simulink library "cyclopsLib"  (R2020a)
settings: Solver=VariableStepAuto  StartTime=0.0  StopTime=10.0  RelTol=1e-3
values from neighbouring files (symbols this model uses):
  agc_delay_lag = 32    [rev0BB_setup.m]
  agc_detector_coef = ones(1,agc_detector_taps)./agc_detector_taps    [rev0BB_setup.m]
  agc_sat_low = -agcSaturation    (= -12)    [rev0BB_setup.m]
  agc_sat_up = agcSaturation    (= 12)    [rev0BB_setup.m]
  agcDesired = 0    [rev0BB_setup.m]
  agcExpDomain = agcSaturation    (= 12)    [rev0BB_setup.m]
  agcExpResolution = 2^-3    (= 0.125)    [rev0BB_setup.m]
  agcPwrAvgNum = 128    [rev0BB_setup.m]
  agcSettleThresh = 0.65    [rev0BB_setup.m]
  agcStep = 2^-8    (= 0.00390625)    [rev0BB_setup.m]
  atanDomain = 5    [rev0BB_setup.m]
  atanResolution = 2^-9    (= 0.001953125)    [rev0BB_setup.m]
  bitsPerSymbolHeader = log2(radixHeader)    [rev0BB_setup.m]
  bitsPerSymbolMax = log2(radixMax)    [rev0BB_setup.m]
  cefEarlyWarning = 256    [rev0BB_setup.m]
  cefLen = length(x_CEF)    [rev0BB_setup.m]
  coarseCFOAdaptDelay = 1    [rev0BB_setup.m]
  cr_i = 0.020    (= 0.02)    [rev0BB_setup.m]
  cr_i_preamp = 2^-9    (= 0.001953125)    [rev0BB_setup.m]
  cr_int1_sat_low = -cr_integrator1_saturation    (= -0.6)    [rev0BB_setup.m]
  cr_int1_sat_up = cr_integrator1_saturation    (= 0.6)    [rev0BB_setup.m]
  cr_integrator1_decay = 1    [rev0BB_setup.m]
  cr_integrator1_saturation = 0.6    [rev0BB_setup.m]
  cr_mult_pipeline = 1    [rev0BB_setup.m]
  cr_p = 0.015    [rev0BB_setup.m]
  cr_sat2_low = -cr_saturation2    (= -0.6)    [rev0BB_setup.m]
  cr_sat2_up = cr_saturation2    (= 0.6)    [rev0BB_setup.m]
  cr_smooth_num = (1/cr_smooth_samples).*ones(1, cr_smooth_samples)    [rev0BB_setup.m]
  D_32 = [ 1,  4,  8,  2, 16]    [golay.m]    (also in rev0BB_setup.m)
  dataLenSymbols = header_len_bytes*8/bitsPerSymbolHeader + frame_len_bytes*8/bitsPerSymbol    [rev0BB_setup.m]
  delayToOutputFromDataFSM = lmsEqDepth/2-1 + regular_pipeline*9 + cr_mult_pipeline*4    (= 31)    [rev0BB_setup.m]
  enableTRFreqCorrection = true    [rev0BB_setup.m]
  expDomain = 3.3    [rev0BB_setup.m]
  expResolution = 2^-5    (= 0.03125)    [rev0BB_setup.m]
  expTol = .1    (= 0.1)    [rev0BB_setup.m]
  forceSlowRxStrobed = false    [rev0BB_setup.m]
  frac_lut_domain_cr = 64    [rev0BB_setup.m]
  frac_lut_range_max_coarse_cfo = 127    [rev0BB_setup.m]
  frac_lut_range_max_cr = 127    [rev0BB_setup.m]
  frac_lut_range_min_coarse_cfo = -frac_lut_range_max_coarse_cfo    (= -127)    [rev0BB_setup.m]
  frac_lut_range_min_cr = -frac_lut_range_max_cr    (= -127)    [rev0BB_setup.m]
  frac_lut_table_breaks_coarse_cfo = -frac_lut_domain_coarse_cfo:frac_lut_res_coarse_cfo:(frac_lut_domain_coarse_cfo-1)    [rev0BB_setup.m]
  frac_lut_table_breaks_cr = -frac_lut_domain_cr:frac_lut_res_cr:(frac_lut_domain_cr-1)    [rev0BB_setup.m]
  frac_lut_table_data_coarse_cfo = 1./frac_lut_table_breaks_coarse_cfo    [rev0BB_setup.m]
  frac_lut_table_data_cr = 1./frac_lut_table_breaks_cr    [rev0BB_setup.m]
  golay_type = 32    [rev0BB_setup.m]
  header_len_bytes = 8    [rev0BB_setup.m]
  lmsEqDepth = 38    [rev0BB_setup.m]
  lmsStep_init = 0.012    [rev0BB_setup.m]
  lmsStep_meta = (lmsStep_final - lmsStep_init)/cefLen    [rev0BB_setup.m]
  lnDomain = 16    [rev0BB_setup.m]
  lnResolution = 2^-3    (= 0.125)    [rev0BB_setup.m]
  minSTFPeaks = 3    [rev0BB_setup.m]
  mod_scheme_len_bytes = 1    [rev0BB_setup.m]
  modBPS = [1, 2, 4]    [rev0BB_setup.m]
  modKeys = [0, 1, 2]    [rev0BB_setup.m]
  mult_pipeline = 1    [rev0BB_setup.m]
  overSample = 4    [berCurve.m]    (also in rev0BB_setup.m)
  overSamplePer = 1/overSampleFreq    (= 1.25e-08)    [rev0BB_setup.m]
  qam16_demod_scale_factor = qam16_hdl_distance/qam16_power_normalized_distance    [rev0BB_setup.m]
  rcRxFilt = rcSqrtFilt    [rev0BB_setup.m]
  rcTxFilt = rcSqrtFilt    [rev0BB_setup.m]
  regular_pipeline = 1    [rev0BB_setup.m]
  rx_gain = 1    [rev0BB_setup.m]
  rx_gain_i = 1    [rev0BB_setup.m]
  rx_gain_q = 1    [rev0BB_setup.m]
  RxFeedbackPipelining = 128*3    (= 384)    [rev0BB_setup.m]
  stfLen = length(x_STF)    [rev0BB_setup.m]
  timing_differentiator_grpDelay_roundUp = ceil((timing_differentiator_len)/2)    [rev0BB_setup.m]
  timing_integrator1_decay = 0.999    [rev0BB_setup.m]
  timing_p = -1/2^2 -1/2^3    (= -0.375)    [rev0BB_setup.m]
  timing_tolerance = 4    [rev0BB_setup.m]
  timingRecoveryDoneSamplesEarly = 1    [rev0BB_setup.m]
  timingRecoveryDoneSamplesEarlyExtraDelay = -timingRecoveryDoneSamplesEarly+1    (= 0)    [rev0BB_setup.m]
  tr_int1_sat_low = -timing_integrate1_saturate    (= -0.0025)    [rev0BB_setup.m]
  tr_int1_sat_up = timing_integrate1_saturate    (= 0.0025)    [rev0BB_setup.m]
  tr_sat2_low = -timing_saturate2    (= -0.005)    [rev0BB_setup.m]
  tr_sat2_up = timing_saturate2    (= 0.005)    [rev0BB_setup.m]
  trigger = 0.40    (= 0.4)    [rev0BB_setup.m]
  trigger_tolerance = 0.35    [rev0BB_setup.m]
  W_32 = [-1,  1, -1,  1, -1]    [golay.m]    (also in rev0BB_setup.m)
  x_STFRepCount = nSpectrum_STFRepCount_short    (= 60)    [rev0BB_setup.m]
undefined symbols (not defined in the file or in its folder): agc_on, cr_integrator2_saturation, Fast_Rx_Partition, Fast_Slim_Rx_Partition, Feedback_Pipeline, freeze_en_agc, freeze_en_cr_int1, freeze_en_cr_int2, freeze_en_cr_phase, freeze_en_tr_int1, freeze_en_tr_int2, freeze_en_tr_phase, freeze_on_cef_done, freeze_on_stf_done, freeze_on_valid, i, post_cr_i_offset, post_cr_q_offset, rx_offset_correction_i, rx_offset_correction_q, Slow_Rx_Partition, timing_i, timing_i_pre_scale
libraries: simulink x62, helperLib x48, golayLib x15, commdigbbndpm3 x8, commdigbbndam3 x4, commfilt2 x3, hdlsllib x2, dspfdesign x1, simulink_need_slupdate x1, dspsigops x1, dsphdlsigops x1, $bdroot x1
(part 3 of 5)

== system cyclopsLib/cyclops_rx_combined/fast_rx/fast_rx_baseband_slim_encapsulated/slim_fast_rx/AGC/ln1 ==
  note: Note that output type is scaled back
  note: Bound Protection
  In : Inport
  data_type : Inport  Port=2
  Compare To Constant1 : simulink/Logic and Bit Operations/Compare To Constant  relop=>=  const=lnDomain  OutDataTypeStr=boolean
  Compare To Constant4 : simulink/Logic and Bit Operations/Compare To Constant  relop=<=  const=lnResolution  OutDataTypeStr=boolean
  Constant11 : Constant  Value=lnResolution  OutDataTypeStr=Inherit: Inherit via back propagation  SampleTime=-1
  Constant3 : Constant  Value=log(lnDomain)  OutDataTypeStr=Inherit: Inherit via back propagation  SampleTime=-1
  Constant4 : Constant  Value=log(lnResolution)  OutDataTypeStr=Inherit: Inherit via back propagation  SampleTime=-1
  Data Type Duplicate : DataTypeDuplicate
  Data Type Conversion : DataTypeConversion  OutDataTypeStr=single
  Logical Operator : Logic  Operator=OR  AllPortsSameDT=off  OutDataTypeStr=boolean
  Switch2 : Switch  Criteria=u2 ~= 0  OutDataTypeStr=Inherit: Inherit via back propagation
  Switch3 : Switch  Criteria=u2 ~= 0  OutDataTypeStr=Inherit: Inherit via back propagation
  Switch8 : Switch  Criteria=u2 ~= 0  OutDataTypeStr=Inherit: Inherit via back propagation
  ln Lookup Table : Lookup_n-D  NumberOfTableDimensions=1  BreakpointsForDimension1=[lnResolution:lnResolution:lnDomain]  IndexSearchMethod=Evenly spaced points  Table=log([lnResolution:lnResolution:lnDomain])  InterpMethod=Flat  DiagnosticForOutOfRangeInput=Error  RemoveProtectionInput=on  InternalRulePriority=Speed  OutDataTypeStr=Inherit: Inherit via back propagation  RndMeth=Simplest  InputSameDT=on
  Out : Outport  VectorParamsAs1DForOutWhenUnconnected=off
  wires:
  ln Lookup Table/1 -> Switch2/3, Data Type Duplicate/2
  Compare To Constant4/1 -> Switch3/2, Logical Operator/2
  Compare To Constant1/1 -> Switch2/2, Logical Operator/1
  Constant11/1 -> Switch8/1
  Logical Operator/1 -> Switch8/2
  Switch3/1 -> Out/1
  Constant4/1 -> Switch3/1
  Switch2/1 -> Switch3/3
  Constant3/1 -> Switch2/1
  Data Type Conversion/1 -> ln Lookup Table/1
  In/1 -> Compare To Constant4/1, Compare To Constant1/1, Switch8/3
  data_type/1 -> Data Type Duplicate/1
  Switch8/1 -> Data Type Conversion/1

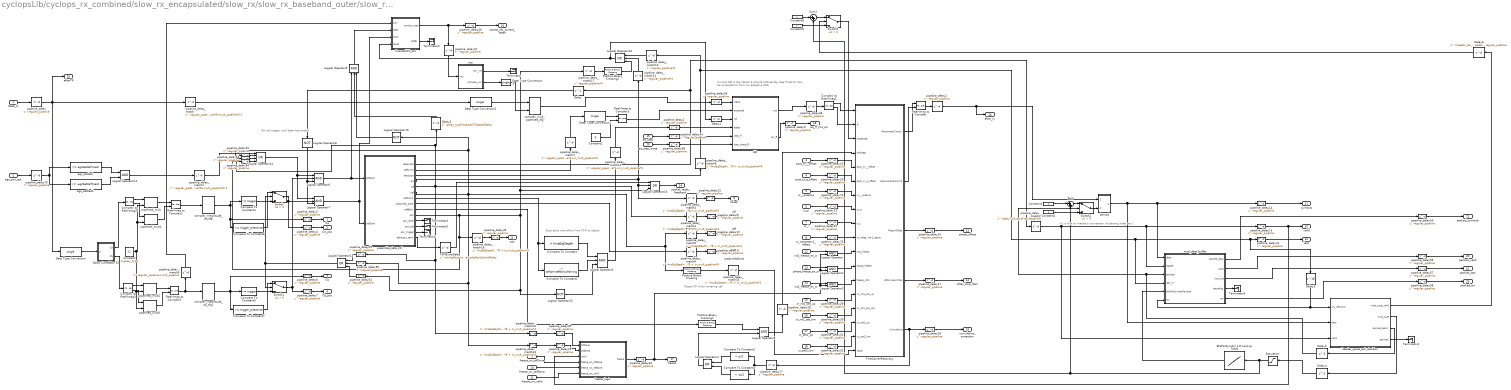
== system cyclopsLib/cyclops_rx_combined/slow_rx_encapsulated/slow_rx/slow_rx_baseband_outer/slow_rx_baseband_enabled/slow_rx_baseband ==
  note: +1 is due to matlab's convention of starting index at 1
  note: Reset CR when entering cef
  note: Current EQ is the classic & simple LMS-LE Alg (see Proakis)
      | Can be extended to form an adaptive DFE
  note: Stop early and allow Fine CFO to adjust
  note: Do not trigger until data has ended
  Data_In : Inport
  agc_pwr_est : Inport  Port=2
  post_cr_i_offset : Inport  Port=3
  post_cr_q_offset : Inport  Port=4
  cr_i_preamp : Inport  Port=5
  cr_p : Inport  Port=6
  cr_i : Inport  Port=7
  cr_integrator1_decay : Inport  Port=8
  freeze_on_stfDone : Inport  Port=9
  freeze_on_cefDone : Inport  Port=10
  freeze_on_valid : Inport  Port=11
  int2_freeze_en_cr : Inport  Port=12  OutDataTypeStr=boolean
  phase_freeze_en_cr : Inport  Port=13  OutDataTypeStr=boolean
  int1_freeze_en_cr : Inport  Port=14  OutDataTypeStr=boolean
  cr_int1_sat_up : Inport  Port=15
  cr_int1_sat_low : Inport  Port=16
  cr_sat2_up : Inport  Port=17
  cr_sat2_low : Inport  Port=18
  eq_step : Inport  Port=19
  eq_step_meta : Inport  Port=20
  " BitsPerSymbol 1-D Lookup Table" : Lookup_n-D  NumberOfTableDimensions=1  BreakpointsForDimension1=modKeys  IndexSearchMethod=Evenly spaced points  Table=modBPS  InterpMethod=Flat  DiagnosticForOutOfRangeInput=Error  InternalRulePriority=Speed  RndMeth=Simplest  InputSameDT=on
  CoarseCFO_est : Subsystem  TreatAsAtomicUnit=on
  Compare To Constant : simulink/Logic and Bit Operations/Compare To Constant  relop=>  const=lmsEqDepth  OutDataTypeStr=boolean
  Compare To Constant1 : simulink/Logic and Bit Operations/Compare To Constant  relop=<  const=cefLen-cefEarlyWarning  OutDataTypeStr=boolean
  Compare To Constant2 : simulink/Logic and Bit Operations/Compare To Constant  relop=>  const=pi/2  OutDataTypeStr=boolean
  Compare To Constant3 : simulink/Logic and Bit Operations/Compare To Constant  relop=<  const=-pi/2  OutDataTypeStr=boolean
  Compare To Constant4 : simulink/Logic and Bit Operations/Compare To Constant  relop=>=  const=trigger  OutDataTypeStr=boolean
  Compare To Constant5 : simulink/Logic and Bit Operations/Compare To Constant  relop=>=  const=trigger  OutDataTypeStr=boolean
  Compare To Constant6 : simulink/Logic and Bit Operations/Compare To Constant  relop=>=  const=trigger_tolerance  OutDataTypeStr=boolean
  Compare To Constant7 : simulink/Logic and Bit Operations/Compare To Constant  relop=>=  const=trigger_tolerance  OutDataTypeStr=boolean
  Complex to Real-Imag1 : ComplexToRealImag
  Complex to Real-Imag2 : ComplexToRealImag
  Complex to Real-Imag3 : ComplexToRealImag
  Constant : Constant  Value=1/golay_type  OutDataTypeStr=Inherit: Inherit via back propagation  SampleTime=-1
  Constant1 : Constant  Value=0  OutDataTypeStr=Inherit: Inherit via back propagation  SampleTime=-1
  Constant{2..3,5..6} (4 alike) : Constant  OutDataTypeStr=uint8  SampleTime=-1
  Data Type Conversion{,1..3} (4 alike) : DataTypeConversion  OutDataTypeStr=single
  Delay : Delay  DelayLength=1  InitialCondition=0
  Delay1 : Delay  InitialCondition=0
  Delay2 : Delay  DelayLength=golay_type*coarseCFOAdaptDelay
  Delay3 : Delay  DelayLength=16
  Delay4 : Delay  DelayLength=1
  Delay5 : Delay  DelayLength=1
  Delay6 : Delay  DelayLength=(header_len_bytes-mod_scheme_len_bytes)*8/bitsPerSymbolHeader - regular_pipeline
  EQ : Subsystem  TreatAsAtomicUnit=on
  FSMExtraDelay : Delay  DelayLength=timingRecoveryDoneSamplesEarlyExtraDelay
  FineCarrierRecovery : Subsystem  TreatAsAtomicUnit=on
  Golay Correlator 32 : Subsystem  TreatAsAtomicUnit=on
  Logical Operator{,1..2,5,11} (5 alike) : Logic  AllPortsSameDT=off  OutDataTypeStr=boolean
  Logical Operator10 : Logic  Operator=OR  Inputs=3  AllPortsSameDT=off  OutDataTypeStr=boolean
  Logical Operator12 : Logic  Operator=NOT  AllPortsSameDT=off  OutDataTypeStr=boolean
  Logical Operator13 : Logic  Operator=OR  Inputs=3  AllPortsSameDT=off  OutDataTypeStr=boolean
  Logical Operator14 : Logic  Operator=OR  Inputs=4  AllPortsSameDT=off  OutDataTypeStr=boolean
  Logical Operator15 : Logic  Operator=NOT  AllPortsSameDT=off  OutDataTypeStr=boolean
  Logical Operator16 : Logic  Operator=OR  Inputs=3  AllPortsSameDT=off  OutDataTypeStr=boolean
  Logical Operator{3,6..7,9} (4 alike) : Logic  Inputs=3  AllPortsSameDT=off  OutDataTypeStr=boolean
  Logical Operator4 : Logic  Operator=OR  AllPortsSameDT=off  OutDataTypeStr=boolean
  Logical Operator8 : Logic  Operator=NOT  AllPortsSameDT=off  OutDataTypeStr=boolean
  Positive Binary Crossing : helperLib/Positive Binary Crossing  SystemSampleTime=-1  Latency=0  AutoFrameSizeCalculation=off
  Positive Binary Crossing1 : helperLib/Positive Binary Crossing  SystemSampleTime=-1  Latency=0  AutoFrameSizeCalculation=off
  Positive Binary Crossing2 : helperLib/Positive Binary Crossing  SystemSampleTime=-1  Latency=0  AutoFrameSizeCalculation=off
  Real-Imag to Complex{,1..3} (4 alike) : RealImagToComplex
  Saturation : Saturate  UpperLimit=modKeys(length(modKeys))  LowerLimit=modKeys(1)
  Sum : Sum  Inputs=|++  OutDataTypeStr=Inherit: Inherit via back propagation
  Sum2 : Sum  Inputs=|++  OutDataTypeStr=Inherit: Inherit via back propagation
  Switch{,1..3} (4 alike) : Switch  Criteria=u2 > Threshold
  Terminator{,1..6} (7 alike) : Terminator
  agc_settled : simulink/Logic and Bit Operations/Compare To Constant  relop=<=  const=agcSettleThresh  OutDataTypeStr=boolean
  agc_settled1 : simulink/Logic and Bit Operations/Compare To Constant  relop=>=  const=-agcSettleThresh  OutDataTypeStr=boolean
  complex_magnitude_sq_cfg : helperLib/complex_magnitude_sq_cfg  mult=mult_pipeline  pipe=regular_pipeline
  complex_magnitude_sq_cfg1 : helperLib/complex_magnitude_sq_cfg  mult=mult_pipeline  pipe=regular_pipeline
  complex_mult_pipelined_cfg : helperLib/complex_mult_pipelined_cfg  mult=cr_mult_pipeline  pipe=regular_pipeline
  demod : Subsystem
  freeze_logic : Subsystem  TreatAsAtomicUnit=on
  header_parse_ack_decision : Subsystem  TreatAsAtomicUnit=on
  mod_data_buffer : Subsystem  TreatAsAtomicUnit=on
  nco : Subsystem  TreatAsAtomicUnit=on
  pipeline_delay{,1..7,9..40,45,49..58} (51 alike) : Delay  DelayLength=regular_pipeline
  pipeline_delay_match : Delay  DelayLength=regular_pipeline*8+mult_pipeline*2-1
  pipeline_delay_match1 : Delay  DelayLength=regular_pipeline*8+mult_pipeline*2-1
  pipeline_delay_match10 : Delay  DelayLength=regular_pipeline*4
  pipeline_delay_match11 : Delay  DelayLength=regular_pipeline*4
  pipeline_delay_match12 : Delay  DelayLength=regular_pipeline*2+cr_mult_pipeline*2
  pipeline_delay_match13 : Delay  DelayLength=lmsEqDepth/2-1 + regular_pipeline*8 + cr_mult_pipeline*4
  pipeline_delay_match14 : Delay  DelayLength=lmsEqDepth/2-1 + regular_pipeline*8 + cr_mult_pipeline*4
  pipeline_delay_match16 : Delay  DelayLength=lmsEqDepth/2-1 + regular_pipeline*5 + cr_mult_pipeline*2
  pipeline_delay_match17 : Delay  DelayLength=regular_pipeline*4
  pipeline_delay_match{3..6,8,18} (6 alike) : Delay  DelayLength=lmsEqDepth/2-1 + regular_pipeline*9 + cr_mult_pipeline*4
  pipeline_delay_match2 : Delay  DelayLength=delayToOutputFromDataFSM
  pipeline_delay_match7 : Delay  DelayLength=regular_pipeline*2+cr_mult_pipeline*2
  pipeline_delay_match9 : Delay  DelayLength=regular_pipeline+mult_pipeline
  pipelined_mult{,1..3} (4 alike) : helperLib/pipelined_mult  d=mult_pipeline
  preamble_data_ctrl : Subsystem  TreatAsAtomicUnit=on
  Ca : Outport  VectorParamsAs1DForOutWhenUnconnected=off
  Ca_pos : Outport  Port=2  VectorParamsAs1DForOutWhenUnconnected=off
  Cb : Outport  Port=3  VectorParamsAs1DForOutWhenUnconnected=off
  Cb_pos : Outport  Port=4  VectorParamsAs1DForOutWhenUnconnected=off
  stf : Outport  Port=5  VectorParamsAs1DForOutWhenUnconnected=off
  cef : Outport  Port=6  VectorParamsAs1DForOutWhenUnconnected=off
  preambleDone : Outport  Port=7  VectorParamsAs1DForOutWhenUnconnected=off
  ack : Outport  Port=8  VectorParamsAs1DForOutWhenUnconnected=off
  failed : Outport  Port=9  VectorParamsAs1DForOutWhenUnconnected=off
  valid : Outport  Port=10  VectorParamsAs1DForOutWhenUnconnected=off
  symbols : Outport  Port=11  VectorParamsAs1DForOutWhenUnconnected=off
  last : Outport  Port=12  VectorParamsAs1DForOutWhenUnconnected=off
  phase_offset : Outport  Port=13  VectorParamsAs1DForOutWhenUnconnected=off
  after_loop_filter : Outport  Port=14  VectorParamsAs1DForOutWhenUnconnected=off
  cumulative_correction : Outport  Port=15  VectorParamsAs1DForOutWhenUnconnected=off
  after_cr : Outport  Port=16  VectorParamsAs1DForOutWhenUnconnected=off
  freeze : Outport  Port=17  VectorParamsAs1DForOutWhenUnconnected=off
  eq_ff_lms_err : Outport  Port=18  VectorParamsAs1DForOutWhenUnconnected=off
  coarse_cfo_correct_steps : Outport  Port=19  VectorParamsAs1DForOutWhenUnconnected=off
  packed_valid : Outport  Port=20  VectorParamsAs1DForOutWhenUnconnected=off
  packed_symbols : Outport  Port=21  VectorParamsAs1DForOutWhenUnconnected=off
  packed_last : Outport  Port=22  VectorParamsAs1DForOutWhenUnconnected=off
  packed_err : Outport  Port=23  VectorParamsAs1DForOutWhenUnconnected=off
  packet_reset_feedback : Outport  Port=24
  afterTR : Outport  Port=25
  wires:
  preamble_data_ctrl/14(dataLast_early) -> FSMExtraDelay/1
  FSMExtraDelay/1 -> Logical Operator16/1
  Logical Operator16/1 -> packet_reset_feedback/1
  Complex to Real-Imag1/1 -> FineCarrierRecovery/1(I)
  Complex to Real-Imag1/2 -> FineCarrierRecovery/2(Q)
  FineCarrierRecovery/1(Recovered Const I) -> Real-Imag to Complex/1
  FineCarrierRecovery/2(Recovered Const Q) -> Real-Imag to Complex/2
  FineCarrierRecovery/3(Phase Offset) -> pipeline_delay16/1
  FineCarrierRecovery/4(After Loop Filter) -> pipeline_delay17/1
  FineCarrierRecovery/5(Cumulative) -> pipeline_delay27/1, pipeline_delay18/1
  pipeline_delay14/1 -> symbols/1
  pipeline_delay13/1 -> freeze_logic/3(valid), valid/1
  pipeline_delay12/1 -> failed/1
  pipeline_delay11/1 -> preambleDone/1
  pipeline_delay10/1 -> cef/1
  pipeline_delay9/1 -> stf/1
  pipeline_delay7/1 -> Cb_pos/1
  pipeline_delay6/1 -> Cb/1
  pipeline_delay4/1 -> Ca_pos/1
  pipeline_delay3/1 -> Ca/1
  Real-Imag to Complex/1 -> pipeline_delay1/1
  Data_In/1 -> pipeline_delay/1
  pipeline_delay16/1 -> phase_offset/1
  pipeline_delay17/1 -> after_loop_filter/1
  pipeline_delay18/1 -> cumulative_correction/1
  post_cr_i_offset/1 -> pipeline_delay19/1
  post_cr_q_offset/1 -> pipeline_delay20/1
  pipeline_delay19/1 -> FineCarrierRecovery/5(post_cr_i_offset)
  pipeline_delay20/1 -> FineCarrierRecovery/6(post_cr_q_offset)
  cr_i_preamp/1 -> pipeline_delay22/1
  cr_p/1 -> pipeline_delay23/1
  cr_i/1 -> pipeline_delay24/1
  cr_integrator1_decay/1 -> pipeline_delay25/1
  pipeline_delay22/1 -> FineCarrierRecovery/7(cr_i_preamp)
  pipeline_delay23/1 -> FineCarrierRecovery/8(cr_p)
  pipeline_delay24/1 -> FineCarrierRecovery/9(cr_i)
  pipeline_delay25/1 -> FineCarrierRecovery/10(cr_integrator1_decay)
  pipeline_delay33/1 -> Logical Operator2/2, Logical Operator1/2, Logical Operator/2, freeze/1
  freeze_on_stfDone/1 -> freeze_logic/4(freeze_on_stfDone)
  freeze_on_cefDone/1 -> freeze_logic/5(freeze_on_cefDone)
  freeze_on_valid/1 -> freeze_logic/6(freeze_on_valid)
  freeze_logic/1(freeze) -> pipeline_delay33/1
  Logical Operator/1 -> FineCarrierRecovery/11(int2_freeze)
  int2_freeze_en_cr/1 -> Logical Operator/1
  cr_int1_sat_up/1 -> pipeline_delay29/1
  pipeline_delay29/1 -> FineCarrierRecovery/14(cr_int1_sat_up)
  cr_sat2_low/1 -> pipeline_delay32/1
  pipeline_delay32/1 -> FineCarrierRecovery/17(cr_sat2_low)
  cr_sat2_up/1 -> pipeline_delay31/1
  pipeline_delay31/1 -> FineCarrierRecovery/16(cr_sat2_up)
  cr_int1_sat_low/1 -> pipeline_delay30/1
  pipeline_delay30/1 -> FineCarrierRecovery/15(cr_int1_sat_low)
  phase_freeze_en_cr/1 -> Logical Operator1/1
  Logical Operator1/1 -> FineCarrierRecovery/12(phase_freeze)
  Logical Operator2/1 -> FineCarrierRecovery/13(freeze_int1)
  int1_freeze_en_cr/1 -> Logical Operator2/1
  pipeline_delay21/1 -> last/1
  Real-Imag to Complex1/1 -> complex_magnitude_sq_cfg/1
  Golay Correlator 32/1(Ca) -> Complex to Real-Imag2/1
  Complex to Real-Imag2/1 -> pipelined_mult/1
  Complex to Real-Imag2/2 -> pipelined_mult1/1
  pipelined_mult/1 -> Real-Imag to Complex1/1
  pipelined_mult1/1 -> Real-Imag to Complex1/2
  Constant/1 -> pipelined_mult1/2, pipelined_mult/2, pipelined_mult3/2, pipelined_mult2/2
  Complex to Real-Imag3/1 -> pipelined_mult2/1
  Complex to Real-Imag3/2 -> pipelined_mult3/1
  pipelined_mult2/1 -> Real-Imag to Complex2/1
  pipelined_mult3/1 -> Real-Imag to Complex2/2
  Golay Correlator 32/2(Cb) -> Complex to Real-Imag3/1
  Data Type Conversion/1 -> Golay Correlator 32/1(In)
  agc_pwr_est/1 -> pipeline_delay26/1
  pipeline_delay26/1 -> agc_settled/1, agc_settled1/1
  Logical Operator6/1 -> preamble_data_ctrl/1(stfStart), Logical Operator9/1
  Logical Operator7/1 -> CoarseCFO_est/3(stop), preamble_data_ctrl/2(cefStart)
  Logical Operator11/1 -> pipeline_delay_match1/1
  Data Type Conversion1/1 -> Real-Imag to Complex3/1
  Constant1/1 -> Real-Imag to Complex3/2
  pipeline_delay_match/1 -> Data Type Conversion2/1
  Compare To Constant/1 -> Logical Operator3/1
  Compare To Constant1/1 -> Logical Operator3/2
  Logical Operator3/1 -> pipeline_delay_match12/1
  Compare To Constant2/1 -> Logical Operator4/1
  Compare To Constant3/1 -> Logical Operator4/2
  pipeline_delay27/1 -> Compare To Constant3/1, Compare To Constant2/1
  Logical Operator4/1 -> Logical Operator5/2
  Positive Binary Crossing1/1 -> Logical Operator5/1
  Logical Operator5/1 -> pipeline_delay28/1
  pipeline_delay28/1 -> FineCarrierRecovery/4(Shift180)
  demod/1(Out1) -> pipeline_delay14/1, mod_data_buffer/1(data), header_parse_ack_decision/2(data)
  pipeline_delay_match3/1 -> pipeline_delay12/1
  pipeline_delay_match6/1 -> pipeline_delay11/1
  pipeline_delay_match5/1 -> pipeline_delay10/1
  pipeline_delay_match4/1 -> pipeline_delay9/1
  Logical Operator8/1 -> Logical Operator6/3, Logical Operator7/3
  Delay/1 -> Logical Operator8/1
  eq_step/1 -> pipeline_delay34/1
  pipeline_delay/1 -> Data Type Conversion/1, pipeline_delay_match/1, afterTR/1
  pipeline_delay36/1 -> Complex to Real-Imag1/1
  Real-Imag to Complex2/1 -> complex_magnitude_sq_cfg1/1, pipeline_delay_match9/1
  Logical Operator9/1 -> CoarseCFO_est/2(peak)
  pipeline_delay_match10/1 -> Logical Operator10/1
  Logical Operator10/1 -> CoarseCFO_est/4(reset), Delay1/1
  pipeline_delay_match9/1 -> CoarseCFO_est/1(corr)
  CoarseCFO_est/1(correct_step) -> pipeline_delay40/1, pipeline_delay37/1
  complex_mult_pipelined_cfg/1 -> pipeline_delay35/1
  pipeline_delay_match11/1 -> Logical Operator10/2
  pipeline_delay_match7/1 -> Data Type Conversion1/1
  Real-Imag to Complex3/1 -> EQ/2(expected)
  Delay1/1 -> EQ/3(rst)
  pipeline_delay_match12/1 -> pipeline_delay2/1
  pipeline_delay34/1 -> EQ/5(step_ff)
  EQ/1(out) -> pipeline_delay36/1
  EQ/2(err_ff) -> pipeline_delay5/1
  pipeline_delay35/1 -> EQ/1(signal)
  agc_settled/1 -> Logical Operator11/1
  agc_settled1/1 -> Logical Operator11/2
  eq_step_meta/1 -> pipeline_delay38/1
  pipeline_delay38/1 -> EQ/6(step_meta_ff)
  pipeline_delay_match13/1 -> pipeline_delay15/1
  pipeline_delay_match14/1 -> pipeline_delay39/1
  pipeline_delay15/1 -> freeze_logic/2(cefDone)
  pipeline_delay39/1 -> freeze_logic/1(stfDone)
  pipeline_delay5/1 -> eq_ff_lms_err/1
  pipeline_delay40/1 -> coarse_cfo_correct_steps/1
  CoarseCFO_est/2(buffer) -> Terminator2/1
  preamble_data_ctrl/6(cef) -> pipeline_delay50/1, pipeline_delay_match13/1, Positive Binary Crossing/1, pipeline_delay_match5/1, Logical Operator15/1, pipeline_delay53/1
  preamble_data_ctrl/4(err) -> pipeline_delay_match11/1, Logical Operator16/2, pipeline_delay_match3/1
  preamble_data_ctrl/7(cefCount) -> Compare To Constant/1, Compare To Constant1/1
  preamble_data_ctrl/2(cefSymb) -> pipeline_delay_match7/1
  preamble_data_ctrl/3(dataLast) -> pipeline_delay_match8/1
  preamble_data_ctrl/8(preamble_done) -> pipeline_delay_match6/1
  preamble_data_ctrl/9(cefEarly) -> Positive Binary Crossing1/1
  nco/1(incr_int) -> Terminator/1
  Positive Binary Crossing/1 -> pipeline_delay_match16/1
  pipeline_delay_match16/1 -> FineCarrierRecovery/18(reset)
  Logical Operator12/1 -> Logical Operator3/3
  Positive Binary Crossing2/1 -> Logical Operator10/3
  pipeline_delay_match17/1 -> Positive Binary Crossing2/1
  preamble_data_ctrl/10(ack) -> Logical Operator16/3, pipeline_delay_match17/1, pipeline_delay51/1, Logical Operator12/1, pipeline_delay54/1, pipeline_delay_match18/1
  pipeline_delay45/1 -> ack/1
  pipeline_delay_match18/1 -> pipeline_delay45/1
  Logical Operator14/1 -> Logical Operator7/1, Logical Operator6/1
  pipeline_delay2/1 -> EQ/4(adapt)
  complex_magnitude_sq_cfg/1 -> Compare To Constant4/1, Compare To Constant6/1, pipeline_delay3/1
  Switch/1 -> pipeline_delay4/1, Logical Operator7/2
  complex_magnitude_sq_cfg1/1 -> Compare To Constant7/1, Compare To Constant5/1, pipeline_delay6/1
  Switch1/1 -> pipeline_delay7/1, Logical Operator6/2
  Compare To Constant4/1 -> Switch/3
  Compare To Constant5/1 -> Switch1/3
  Compare To Constant7/1 -> Switch1/1
  Compare To Constant6/1 -> Switch/1
  Logical Operator13/1 -> Switch/2, Switch1/2
  pipeline_delay49/1 -> Logical Operator13/1
  pipeline_delay50/1 -> Logical Operator13/2
  pipeline_delay51/1 -> Logical Operator13/3
  pipeline_delay_match1/1 -> Logical Operator14/1
  pipeline_delay52/1 -> Logical Operator14/2
  pipeline_delay53/1 -> Logical Operator14/3
  pipeline_delay54/1 -> Logical Operator14/4
  Data Type Conversion2/1 -> complex_mult_pipelined_cfg/1
  nco/2(complex_sin) -> Data Type Conversion3/1
  preamble_data_ctrl/5(stf) -> pipeline_delay49/1, pipeline_delay_match14/1, pipeline_delay_match4/1, Delay2/1, pipeline_delay52/1
  Delay2/1 -> Logical Operator9/2
  Logical Operator15/1 -> Logical Operator9/3
  pipeline_delay_match2/1 -> mod_data_buffer/2(header), pipeline_delay13/1, header_parse_ack_decision/3(valid)
  Switch3/1 -> FineCarrierRecovery/3(ModMode)
  header_parse_ack_decision/3(payload_early) -> Delay5/1
  header_parse_ack_decision/2(mod_type) -> Delay4/1
  Delay4/1 -> Saturation/1
  " BitsPerSymbol 1-D Lookup Table"/1 -> mod_data_buffer/5(bitsPerSymbolPayload)
  Switch2/1 -> demod/2(ModMode)
  Constant2/1 -> Switch2/3
  Sum/1 -> Switch2/1
  Constant3/1 -> Sum/1
  Sum2/1 -> Switch3/1
  Constant6/1 -> Sum2/1
  Constant5/1 -> Switch3/3
  Delay3/1 -> header_parse_ack_decision/1(crc_decision), mod_data_buffer/6(rst)
  mod_data_buffer/1(packed_data) -> pipeline_delay56/1
  mod_data_buffer/2(valid) -> pipeline_delay55/1
  pipeline_delay56/1 -> packed_symbols/1
  pipeline_delay55/1 -> packed_valid/1
  pipeline_delay57/1 -> packed_last/1
  mod_data_buffer/3(last_out) -> pipeline_delay57/1
  pipeline_delay_match8/1 -> mod_data_buffer/4(last_in), Delay3/1, pipeline_delay21/1, pipeline_delay_match10/1
  preamble_data_ctrl/1(dataValid) -> Delay/1, pipeline_delay_match2/1
  pipeline_delay1/1 -> after_cr/1, demod/1(In1)
  Delay5/1 -> mod_data_buffer/3(payload), Switch2/2
  header_parse_ack_decision/4(payload) -> Terminator1/1
  header_parse_ack_decision/1(mod_type_valid) -> Delay6/1
  Delay6/1 -> Switch3/2
  pipeline_delay58/1 -> packed_err/1
  mod_data_buffer/5(err) -> pipeline_delay58/1
  Data Type Conversion3/1 -> complex_mult_pipelined_cfg/2
  pipeline_delay37/1 -> nco/1(incr)
  Saturation/1 -> " BitsPerSymbol 1-D Lookup Table"/1, Sum/2, Sum2/2
  mod_data_buffer/4(decoding) -> Terminator3/1
  preamble_data_ctrl/11(ack_done) -> Terminator4/1
  preamble_data_ctrl/12(ack_dst) -> Terminator5/1
  preamble_data_ctrl/13(ack_trigger) -> Terminator6/1

== system cyclopsLib/cyclops_rx_combined/fast_rx/fast_rx_baseband_encapsulated/fast_rx_baseband/Timing Recovery/cefEarlyWarning/Golay Correlator 32 ==
  In : Inport
  GolayCoralatorBase_fp : golayLib/GolayCoralatorBase_fp  dSub=D_32(1)*4  wSub=W_32(1)  mult=0
  GolayCoralatorBase_fp1 : golayLib/GolayCoralatorBase_fp  dSub=D_32(2)*4  wSub=W_32(2)  mult=0
  GolayCoralatorBase_fp2 : golayLib/GolayCoralatorBase_fp  dSub=D_32(3)*4  wSub=W_32(3)  mult=0
  GolayCoralatorBase_fp3 : golayLib/GolayCoralatorBase_fp  dSub=D_32(4)*4  wSub=W_32(4)  mult=0
  GolayCoralatorBase_fp4 : golayLib/GolayCoralatorBase_fp  dSub=D_32(5)*4  wSub=W_32(5)  mult=0
  pipeline_delay{,1..13} (14 alike) : Delay  DelayLength=regular_pipeline
  Ca : Outport  VectorParamsAs1DForOutWhenUnconnected=off
  Cb : Outport  Port=2  VectorParamsAs1DForOutWhenUnconnected=off
  wires:
  pipeline_delay11/1 -> pipeline_delay13/1
  GolayCoralatorBase_fp4/2 -> pipeline_delay9/1
  pipeline_delay7/1 -> GolayCoralatorBase_fp4/2
  pipeline_delay5/1 -> GolayCoralatorBase_fp3/2
  pipeline_delay13/1 -> Cb/1
  pipeline_delay12/1 -> Ca/1
  pipeline_delay6/1 -> GolayCoralatorBase_fp4/1
  pipeline_delay4/1 -> GolayCoralatorBase_fp3/1
  pipeline_delay3/1 -> GolayCoralatorBase_fp2/2
  pipeline_delay2/1 -> GolayCoralatorBase_fp2/1
  pipeline_delay1/1 -> GolayCoralatorBase_fp1/2
  pipeline_delay/1 -> GolayCoralatorBase_fp1/1
  In/1 -> GolayCoralatorBase_fp/1, GolayCoralatorBase_fp/2
  pipeline_delay10/1 -> pipeline_delay12/1
  pipeline_delay8/1 -> pipeline_delay10/1
  pipeline_delay9/1 -> pipeline_delay11/1
  GolayCoralatorBase_fp3/2 -> pipeline_delay7/1
  GolayCoralatorBase_fp3/1 -> pipeline_delay6/1
  GolayCoralatorBase_fp2/2 -> pipeline_delay5/1
  GolayCoralatorBase_fp2/1 -> pipeline_delay4/1
  GolayCoralatorBase_fp4/1 -> pipeline_delay8/1
  GolayCoralatorBase_fp1/2 -> pipeline_delay3/1
  GolayCoralatorBase_fp1/1 -> pipeline_delay2/1
  GolayCoralatorBase_fp/2 -> pipeline_delay1/1
  GolayCoralatorBase_fp/1 -> pipeline_delay/1

== system cyclopsLib/cyclops_rx_combined/fast_rx/fast_rx_baseband_encapsulated/fast_rx_baseband/Timing Recovery/correlateAndDetectPhaseError/Golay Correlator 32 ==
  In : Inport
  GolayCoralatorBase_fp : golayLib/GolayCoralatorBase_fp  dSub=D_32(1)*4  wSub=W_32(1)  mult=0
  GolayCoralatorBase_fp1 : golayLib/GolayCoralatorBase_fp  dSub=D_32(2)*4  wSub=W_32(2)  mult=0
  GolayCoralatorBase_fp2 : golayLib/GolayCoralatorBase_fp  dSub=D_32(3)*4  wSub=W_32(3)  mult=0
  GolayCoralatorBase_fp3 : golayLib/GolayCoralatorBase_fp  dSub=D_32(4)*4  wSub=W_32(4)  mult=0
  GolayCoralatorBase_fp4 : golayLib/GolayCoralatorBase_fp  dSub=D_32(5)*4  wSub=W_32(5)  mult=0
  pipeline_delay{,1..13} (14 alike) : Delay  DelayLength=regular_pipeline
  Ca : Outport  VectorParamsAs1DForOutWhenUnconnected=off
  Cb : Outport  Port=2  VectorParamsAs1DForOutWhenUnconnected=off
  wires:
  pipeline_delay11/1 -> pipeline_delay13/1
  GolayCoralatorBase_fp4/2 -> pipeline_delay9/1
  pipeline_delay7/1 -> GolayCoralatorBase_fp4/2
  pipeline_delay5/1 -> GolayCoralatorBase_fp3/2
  pipeline_delay13/1 -> Cb/1
  pipeline_delay12/1 -> Ca/1
  pipeline_delay6/1 -> GolayCoralatorBase_fp4/1
  pipeline_delay4/1 -> GolayCoralatorBase_fp3/1
  pipeline_delay3/1 -> GolayCoralatorBase_fp2/2
  pipeline_delay2/1 -> GolayCoralatorBase_fp2/1
  pipeline_delay1/1 -> GolayCoralatorBase_fp1/2
  pipeline_delay/1 -> GolayCoralatorBase_fp1/1
  In/1 -> GolayCoralatorBase_fp/1, GolayCoralatorBase_fp/2
  pipeline_delay10/1 -> pipeline_delay12/1
  pipeline_delay8/1 -> pipeline_delay10/1
  pipeline_delay9/1 -> pipeline_delay11/1
  GolayCoralatorBase_fp3/2 -> pipeline_delay7/1
  GolayCoralatorBase_fp3/1 -> pipeline_delay6/1
  GolayCoralatorBase_fp2/2 -> pipeline_delay5/1
  GolayCoralatorBase_fp2/1 -> pipeline_delay4/1
  GolayCoralatorBase_fp4/1 -> pipeline_delay8/1
  GolayCoralatorBase_fp1/2 -> pipeline_delay3/1
  GolayCoralatorBase_fp1/1 -> pipeline_delay2/1
  GolayCoralatorBase_fp/2 -> pipeline_delay1/1
  GolayCoralatorBase_fp/1 -> pipeline_delay/1

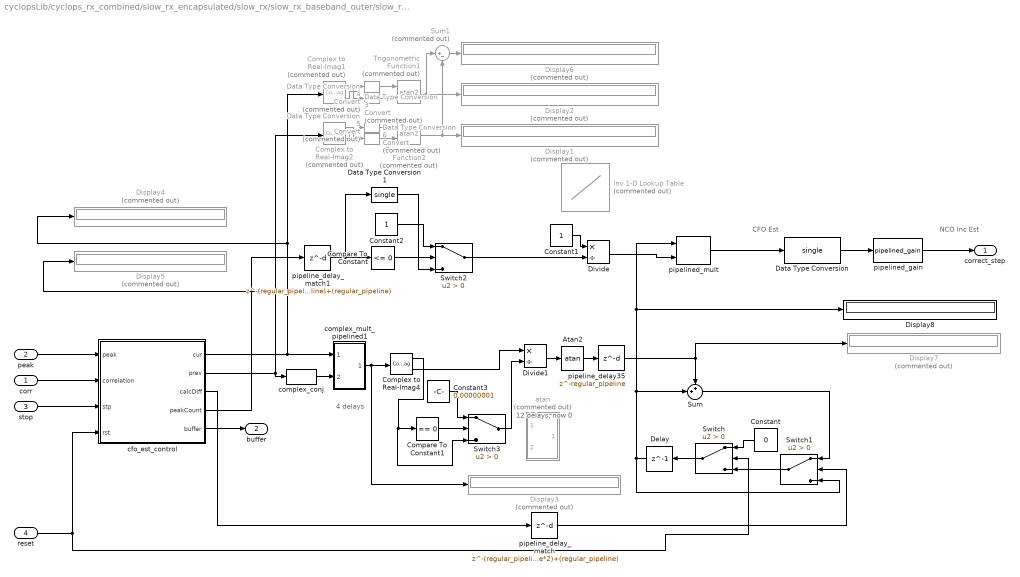
== system cyclopsLib/cyclops_rx_combined/slow_rx_encapsulated/slow_rx/slow_rx_baseband_outer/slow_rx_baseband_enabled/slow_rx_baseband/CoarseCFO_est ==
  note: NCO Inc Est
  note: CFO Est
  note: 4 delays
  note: 12 delays, now 0
  corr : Inport
  peak : Inport  Port=2
  stop : Inport  Port=3
  reset : Inport  Port=4  OutDataTypeStr=boolean
  Atan2 : Trigonometry  Operator=atan
  Compare To Constant : simulink/Logic and Bit Operations/Compare To Constant  relop=<=  const=0  OutDataTypeStr=boolean
  Compare To Constant1 : simulink/Logic and Bit Operations/Compare To Constant  relop===  const=0  OutDataTypeStr=boolean
  Complex to Real-Imag1 : ComplexToRealImag  Commented=on
  Complex to Real-Imag2 : ComplexToRealImag  Commented=on
  Complex to Real-Imag4 : ComplexToRealImag
  Constant : Constant  Value=0  OutDataTypeStr=Inherit: Inherit via back propagation  SampleTime=-1
  Constant1 : Constant  OutDataTypeStr=Inherit: Inherit via back propagation
  Constant2 : Constant  OutDataTypeStr=Inherit: Inherit via back propagation
  Constant3 : Constant  Value=0.00000001  OutDataTypeStr=Inherit: Inherit via back propagation
  Data Type Conversion : DataTypeConversion  OutDataTypeStr=single
  Data Type Conversion1 : DataTypeConversion  OutDataTypeStr=single
  Data Type Conversion{3..6} (4 alike) : DataTypeConversion  Commented=on
  Delay : Delay  DelayLength=1  InitialCondition=0
  Display{1..7} (7 alike) : Display  Commented=on
  Display8 : Display
  Divide : Product  Inputs=*/
  Divide1 : Product  Inputs=*/
  Inv 1-D Lookup Table : Lookup_n-D  Commented=on  NumberOfTableDimensions=1  BreakpointsForDimension1=[0:(x_STFRepCount+1)]  IndexSearchMethod=Evenly spaced points  Table=cat(2, [1], 1./[1:(x_STFRepCount+1)] )  InterpMethod=Flat  DiagnosticForOutOfRangeInput=Error  InternalRulePriority=Speed  OutDataTypeStr=Inherit: Inherit via back propagation  RndMeth=Simplest  InputSameDT=on
  Sum : Sum  Inputs=++|  OutDataTypeStr=Inherit: Same as first input
  Sum1 : Sum  Commented=on  Inputs=|+-
  Switch{,1..3} (4 alike) : Switch  Criteria=u2 > Threshold
  Trigonometric Function1 : Trigonometry  Commented=on  Operator=atan2
  Trigonometric Function2 : Trigonometry  Commented=on  Operator=atan2
  atan : Subsystem  Commented=on  AncestorBlock=helperLib/atan2
  cfo_est_control : Stateflow chart  TreatAsAtomicUnit=on
  complex_conj : helperLib/complex_conj  SystemSampleTime=-1  Latency=0  AutoFrameSizeCalculation=off
  complex_mult_pipelined1 : Subsystem  AncestorBlock=helperLib/complex_mult_pipelined
  pipeline_delay35 : Delay  DelayLength=regular_pipeline
  pipeline_delay_match : Delay  DelayLength=(regular_pipeline*2 + cr_mult_pipeline*2)+(regular_pipeline)
  pipeline_delay_match1 : Delay  DelayLength=(regular_pipeline*2 + cr_mult_pipeline*2)+(regular_pipeline)+(regular_pipeline)
  pipelined_gain : helperLib/pipelined_gain  g=-2^16/(2*pi*golay_type)  d=regular_pipeline
  pipelined_mult : helperLib/pipelined_mult  d=cr_mult_pipeline
  correct_step : Outport  VectorParamsAs1DForOutWhenUnconnected=off
  buffer : Outport  Port=2  VectorParamsAs1DForOutWhenUnconnected=off
  wires:
  complex_mult_pipelined1/1(Out1) -> Complex to Real-Imag4/1, Display3/1
  pipeline_delay35/1 -> Sum/1, Display7/1
  reset/1 -> Switch/2, cfo_est_control/4(rst)
  Sum/1 -> Switch1/1
  cfo_est_control/1(cur) -> Complex to Real-Imag1/1, Display4/1, complex_mult_pipelined1/1(In1)
  complex_conj/1 -> complex_mult_pipelined1/2(In2)
  cfo_est_control/2(prev) -> complex_conj/1, Complex to Real-Imag2/1, Display5/1
  cfo_est_control/4(peakCount) -> pipeline_delay_match1/1
  Switch/1 -> Delay/1
  Switch1/1 -> Switch/3
  Constant/1 -> Switch/1
  cfo_est_control/3(calcDiff) -> pipeline_delay_match/1
  pipeline_delay_match/1 -> Switch1/2
  Data Type Conversion3/1 -> Trigonometric Function1/1
  Data Type Conversion4/1 -> Trigonometric Function1/2
  Complex to Real-Imag1/2 -> Data Type Conversion3/1
  Complex to Real-Imag1/1 -> Data Type Conversion4/1
  Trigonometric Function1/1 -> Sum1/1, Display2/1
  Data Type Conversion5/1 -> Trigonometric Function2/1
  Data Type Conversion6/1 -> Trigonometric Function2/2
  Complex to Real-Imag2/2 -> Data Type Conversion5/1
  Complex to Real-Imag2/1 -> Data Type Conversion6/1
  Trigonometric Function2/1 -> Sum1/2, Display1/1
  Sum1/1 -> Display6/1
  stop/1 -> cfo_est_control/3(stp)
  peak/1 -> cfo_est_control/1(peak)
  corr/1 -> cfo_est_control/2(correlation)
  cfo_est_control/5(buffer) -> buffer/1
  Atan2/1 -> pipeline_delay35/1
  Delay/1 -> Display8/1, pipelined_mult/1, Sum/2, Switch1/3
  pipelined_gain/1 -> correct_step/1
  Data Type Conversion/1 -> pipelined_gain/1
  pipelined_mult/1 -> Data Type Conversion/1
  pipeline_delay_match1/1 -> Data Type Conversion1/1, Compare To Constant/1
  Constant1/1 -> Divide/1
  Compare To Constant/1 -> Switch2/2
  Constant2/1 -> Switch2/1
  Switch2/1 -> Divide/2
  Divide/1 -> pipelined_mult/2
  Complex to Real-Imag4/2 -> Divide1/1
  Divide1/1 -> Atan2/1
  Constant3/1 -> Switch3/1
  Compare To Constant1/1 -> Switch3/2
  Complex to Real-Imag4/1 -> Switch3/3, Compare To Constant1/1
  Switch3/1 -> Divide1/2
  Data Type Conversion1/1 -> Switch2/3

== system cyclopsLib/cyclops_rx_combined/slow_rx_encapsulated/slow_rx/slow_rx_baseband_outer/slow_rx_baseband_enabled/slow_rx_baseband/EQ ==
  signal : Inport
  expected : Inport  Port=2
  rst : Inport  Port=3
  adapt : Inport  Port=4
  step_ff : Inport  Port=5
  step_meta_ff : Inport  Port=6
  Delay : Delay  DelayLength=1  InitialCondition=0
  Display : Display  Commented=on
  Display1 : Display  Commented=on
  Display2 : Display  Commented=on
  Sum : Sum  Inputs=++|  OutDataTypeStr=Inherit: Same as first input
  Switch : Switch  Criteria=u2 > Threshold
  lms : Subsystem  AncestorBlock=helperLib/lms
  out : Outport  VectorParamsAs1DForOutWhenUnconnected=off
  err_ff : Outport  Port=2  VectorParamsAs1DForOutWhenUnconnected=off
  wires:
  adapt/1 -> Switch/2, lms/4(adapt)
  step_ff/1 -> Switch/3, Display/1
  signal/1 -> lms/1(in)
  rst/1 -> lms/3(reset)
  expected/1 -> lms/2(expected)
  lms/2(err) -> err_ff/1
  lms/1(out) -> out/1
  Switch/1 -> Delay/1
  step_meta_ff/1 -> Display1/1, Sum/1
  Delay/1 -> Display2/1, lms/5(step), Sum/2
  Sum/1 -> Switch/1

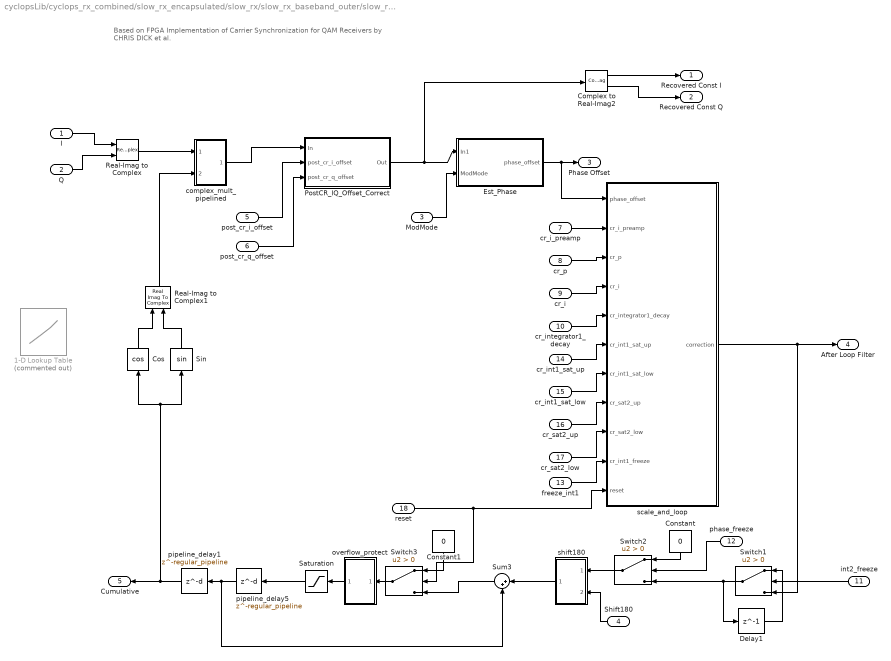
== system cyclopsLib/cyclops_rx_combined/slow_rx_encapsulated/slow_rx/slow_rx_baseband_outer/slow_rx_baseband_enabled/slow_rx_baseband/FineCarrierRecovery ==
  note: Based on FPGA Implementation of Carrier Synchronization for QAM Receivers
      | by CHRIS DICK et al.
  I : Inport  PortDimensions=1
  Q : Inport  Port=2  PortDimensions=1
  ModMode : Inport  Port=3  PortDimensions=1
  Shift180 : Inport  Port=4  OutDataTypeStr=boolean  PortDimensions=1
  post_cr_i_offset : Inport  Port=5
  post_cr_q_offset : Inport  Port=6
  cr_i_preamp : Inport  Port=7
  cr_p : Inport  Port=8
  cr_i : Inport  Port=9
  cr_integrator1_decay : Inport  Port=10
  int2_freeze : Inport  Port=11  OutDataTypeStr=boolean
  phase_freeze : Inport  Port=12  OutDataTypeStr=boolean
  freeze_int1 : Inport  Port=13
  cr_int1_sat_up : Inport  Port=14
  cr_int1_sat_low : Inport  Port=15
  cr_sat2_up : Inport  Port=16
  cr_sat2_low : Inport  Port=17
  reset : Inport  Port=18
  1-D Lookup Table : Lookup_n-D  Commented=on  NumberOfTableDimensions=1  BreakpointsForDimension1=[-expDomain:expResolution:expDomain]  IndexSearchMethod=Evenly spaced points  Table=exp(i*[-expDomain:expResolution:expDomain])  InterpMethod=Flat  DiagnosticForOutOfRangeInput=Error  InternalRulePriority=Speed  RndMeth=Simplest  InputSameDT=on
  Complex to Real-Imag2 : ComplexToRealImag
  Constant : Constant  Value=0  OutDataTypeStr=Inherit: Inherit via back propagation  SampleTime=-1
  Constant1 : Constant  Value=0  OutDataTypeStr=Inherit: Inherit via back propagation  SampleTime=-1
  Cos : Trigonometry  Operator=cos
  Delay1 : Delay  DelayLength=1  InitialCondition=0
  Est_Phase : Subsystem
  PostCR_IQ_Offset_Correct : Subsystem
  Real-Imag to Complex : RealImagToComplex
  Real-Imag to Complex1 : RealImagToComplex
  Saturation : Saturate  UpperLimit=expDomain  LowerLimit=-expDomain
  Sin : Trigonometry
  Sum3 : Sum  Inputs=|++  OutDataTypeStr=Inherit: Same as first input
  Switch1 : Switch  Criteria=u2 > Threshold
  Switch2 : Switch  Criteria=u2 > Threshold
  Switch3 : Switch  Criteria=u2 > Threshold
  complex_mult_pipelined : Subsystem  AncestorBlock=helperLib/complex_mult_pipelined
  overflow_protect : Subsystem
  pipeline_delay1 : Delay  DelayLength=regular_pipeline
  pipeline_delay5 : Delay  DelayLength=regular_pipeline
  scale_and_loop : Subsystem
  shift180 : Subsystem
  Recovered Const I : Outport  PortDimensions=1  VectorParamsAs1DForOutWhenUnconnected=off
  Recovered Const Q : Outport  Port=2  PortDimensions=1  VectorParamsAs1DForOutWhenUnconnected=off
  Phase Offset : Outport  Port=3  PortDimensions=1  VectorParamsAs1DForOutWhenUnconnected=off
  After Loop Filter : Outport  Port=4  PortDimensions=1  VectorParamsAs1DForOutWhenUnconnected=off
  Cumulative : Outport  Port=5  PortDimensions=1  VectorParamsAs1DForOutWhenUnconnected=off
  wires:
  I/1 -> Real-Imag to Complex/1
  Q/1 -> Real-Imag to Complex/2
  shift180/1(Out1) -> Sum3/1
  Real-Imag to Complex1/1 -> complex_mult_pipelined/2(In2)
  Real-Imag to Complex/1 -> complex_mult_pipelined/1(In1)
  Complex to Real-Imag2/1 -> Recovered Const I/1
  Complex to Real-Imag2/2 -> Recovered Const Q/1
  Est_Phase/1(phase_offset) -> scale_and_loop/1(phase_offset), Phase Offset/1
  overflow_protect/1(Out1) -> Saturation/1
  Shift180/1 -> shift180/2(shift180)
  scale_and_loop/1(correction) -> After Loop Filter/1, Switch1/3
  pipeline_delay1/1 -> Cumulative/1, Cos/1, Sin/1
  PostCR_IQ_Offset_Correct/1(Out) -> Complex to Real-Imag2/1, Est_Phase/1(In1)
  complex_mult_pipelined/1(Out1) -> PostCR_IQ_Offset_Correct/1(In)
  post_cr_i_offset/1 -> PostCR_IQ_Offset_Correct/2(post_cr_i_offset)
  post_cr_q_offset/1 -> PostCR_IQ_Offset_Correct/3(post_cr_q_offset)
  cr_i_preamp/1 -> scale_and_loop/2(cr_i_preamp)
  cr_p/1 -> scale_and_loop/3(cr_p)
  cr_i/1 -> scale_and_loop/4(cr_i)
  cr_integrator1_decay/1 -> scale_and_loop/5(cr_integrator1_decay)
  Delay1/1 -> Switch1/1
  int2_freeze/1 -> Switch1/2
  Switch1/1 -> Switch2/3, Delay1/1
  pipeline_delay5/1 -> Sum3/2, pipeline_delay1/1
  cr_int1_sat_up/1 -> scale_and_loop/6(cr_int1_sat_up)
  cr_int1_sat_low/1 -> scale_and_loop/7(cr_int1_sat_low)
  cr_sat2_up/1 -> scale_and_loop/8(cr_sat2_up)
  cr_sat2_low/1 -> scale_and_loop/9(cr_sat2_low)
  phase_freeze/1 -> Switch2/2
  Constant/1 -> Switch2/1
  freeze_int1/1 -> scale_and_loop/10(cr_int1_freeze)
  Switch2/1 -> shift180/1(In1)
  Saturation/1 -> pipeline_delay5/1
  ModMode/1 -> Est_Phase/2(ModMode)
  Switch3/1 -> overflow_protect/1(In1)
  Sum3/1 -> Switch3/3
  Constant1/1 -> Switch3/1
  reset/1 -> Switch3/2, scale_and_loop/11(reset)
  Sin/1 -> Real-Imag to Complex1/2
  Cos/1 -> Real-Imag to Complex1/1

== system cyclopsLib/cyclops_rx_combined/slow_rx_encapsulated/slow_rx/slow_rx_baseband_outer/slow_rx_baseband_enabled/slow_rx_baseband/Golay Correlator 32 ==
  In : Inport
  GolayCoralatorBase_fp : golayLib/GolayCoralatorBase_fp  dSub=D_32(1)  wSub=W_32(1)  mult=0
  GolayCoralatorBase_fp1 : golayLib/GolayCoralatorBase_fp  dSub=D_32(2)  wSub=W_32(2)  mult=0
  GolayCoralatorBase_fp2 : golayLib/GolayCoralatorBase_fp  dSub=D_32(3)  wSub=W_32(3)  mult=0
  GolayCoralatorBase_fp3 : golayLib/GolayCoralatorBase_fp  dSub=D_32(4)  wSub=W_32(4)  mult=0
  GolayCoralatorBase_fp4 : golayLib/GolayCoralatorBase_fp  dSub=D_32(5)  wSub=W_32(5)  mult=0
  pipeline_delay{,1..13} (14 alike) : Delay  DelayLength=regular_pipeline
  Ca : Outport  VectorParamsAs1DForOutWhenUnconnected=off
  Cb : Outport  Port=2  VectorParamsAs1DForOutWhenUnconnected=off
  wires:
  GolayCoralatorBase_fp/1 -> pipeline_delay/1
  GolayCoralatorBase_fp/2 -> pipeline_delay1/1
  GolayCoralatorBase_fp1/1 -> pipeline_delay2/1
  GolayCoralatorBase_fp1/2 -> pipeline_delay3/1
  GolayCoralatorBase_fp4/1 -> pipeline_delay8/1
  GolayCoralatorBase_fp2/1 -> pipeline_delay4/1
  GolayCoralatorBase_fp2/2 -> pipeline_delay5/1
  GolayCoralatorBase_fp3/1 -> pipeline_delay6/1
  GolayCoralatorBase_fp3/2 -> pipeline_delay7/1
  pipeline_delay9/1 -> pipeline_delay11/1
  pipeline_delay8/1 -> pipeline_delay10/1
  pipeline_delay10/1 -> pipeline_delay12/1
  In/1 -> GolayCoralatorBase_fp/2, GolayCoralatorBase_fp/1
  pipeline_delay/1 -> GolayCoralatorBase_fp1/1
  pipeline_delay1/1 -> GolayCoralatorBase_fp1/2
  pipeline_delay2/1 -> GolayCoralatorBase_fp2/1
  pipeline_delay3/1 -> GolayCoralatorBase_fp2/2
  pipeline_delay4/1 -> GolayCoralatorBase_fp3/1
  pipeline_delay6/1 -> GolayCoralatorBase_fp4/1
  pipeline_delay12/1 -> Ca/1
  pipeline_delay13/1 -> Cb/1
  pipeline_delay5/1 -> GolayCoralatorBase_fp3/2
  pipeline_delay7/1 -> GolayCoralatorBase_fp4/2
  GolayCoralatorBase_fp4/2 -> pipeline_delay9/1
  pipeline_delay11/1 -> pipeline_delay13/1

== system cyclopsLib/cyclops_rx_combined/slow_rx_encapsulated/slow_rx/slow_rx_baseband_outer/slow_rx_baseband_enabled/slow_rx_baseband/demod ==
  In1 : Inport
  ModMode : Inport  Port=2
  BPSK Demodulator Baseband : commdigbbndpm3/BPSK Demodulator Baseband  DecType=Hard decision  VarSource=Dialog  Variance=1  Ph=0  outDtype=uint8  derotateFactorWordLen=16  derotateFactorDataTypeStr=Inherit: Same word length as input  derotateFactorLastDataTypeStr=Inherit: Same word length as input
  Gain : Gain  Gain=qam16_demod_scale_factor
  Multiport Switch : MultiPortSwitch
  QPSK Demodulator Baseband : commdigbbndpm3/QPSK Demodulator Baseband  OutType=Integer  DecType=Hard decision  VarSource=Dialog  Variance=1  Dec=Gray  Ph=pi/4  outDtype1=Inherit via internal rule  outDtype2=uint8  derotateFactorWordLen=16  derotateFactorDataTypeStr=Inherit: Same word length as input  derotateFactorLastDataTypeStr=Inherit: Same word length as input
  Rectangular QAM Demodulator Baseband : commdigbbndam3/Rectangular QAM Demodulator Baseband  M=16  OutType=Integer  DecType=Hard decision  VarSource=Dialog  Variance=1  Dec=Gray  Mapping=[0:15]  PowType=Min. distance between symbols  MinDist=qam16_hdl_distance  AvgPow=1  PeakPow=1  Ph=0  outDtype1=Inherit via internal rule  outDtype2=uint8  derotateFactorWordLen=16  derotateFactorDataTypeStr=Inherit: Same word length as input  derotateFactorLastDataTypeStr=Inherit: Same word length as input  denormFactorWordLen=16  denormFactorDataTypeStr=Inherit: Same word length as input  denormFactorLastDataTypeStr=Inherit: Same word length as input  prodOutWordLen=32  prodOutOverflowMode=Wrap  prodOutRoundingMode=Floor  prodOutOvFlMode=off  prodOutOvFlModeLastStrValue=off  sumWordLen=32
  Out1 : Outport  VectorParamsAs1DForOutWhenUnconnected=off
  wires:
  BPSK Demodulator Baseband/1 -> Multiport Switch/2
  In1/1 -> QPSK Demodulator Baseband/1, Gain/1, BPSK Demodulator Baseband/1
  Multiport Switch/1 -> Out1/1
  ModMode/1 -> Multiport Switch/1
  Rectangular QAM Demodulator Baseband/1 -> Multiport Switch/4
  QPSK Demodulator Baseband/1 -> Multiport Switch/3
  Gain/1 -> Rectangular QAM Demodulator Baseband/1

== system cyclopsLib/cyclops_rx_combined/slow_rx_encapsulated/slow_rx/slow_rx_baseband_outer/slow_rx_baseband_enabled/slow_rx_baseband/freeze_logic ==
  stfDone : Inport
  cefDone : Inport  Port=2
  valid : Inport  Port=3
  freeze_on_stfDone : Inport  Port=4  OutDataTypeStr=boolean
  freeze_on_cefDone : Inport  Port=5  OutDataTypeStr=boolean
  freeze_on_valid : Inport  Port=6  OutDataTypeStr=boolean
  Logical Operator : Logic  AllPortsSameDT=off  OutDataTypeStr=boolean
  Logical Operator1 : Logic  AllPortsSameDT=off  OutDataTypeStr=boolean
  Logical Operator3 : Logic  AllPortsSameDT=off  OutDataTypeStr=boolean
  Logical Operator4 : Logic  Operator=OR  Inputs=3  AllPortsSameDT=off  OutDataTypeStr=boolean
  pipeline_delay29 : Delay  DelayLength=regular_pipeline
  pipeline_delay30 : Delay  DelayLength=regular_pipeline
  pipeline_delay32 : Delay  DelayLength=regular_pipeline
  freeze : Outport  OutDataTypeStr=boolean  VectorParamsAs1DForOutWhenUnconnected=off
  wires:
  Logical Operator4/1 -> freeze/1
  freeze_on_cefDone/1 -> pipeline_delay30/1
  freeze_on_valid/1 -> pipeline_delay32/1
  pipeline_delay30/1 -> Logical Operator1/1
  pipeline_delay29/1 -> Logical Operator/1
  valid/1 -> Logical Operator3/2
  cefDone/1 -> Logical Operator1/2
  stfDone/1 -> Logical Operator/2
  Logical Operator1/1 -> Logical Operator4/2
  pipeline_delay32/1 -> Logical Operator3/1
  freeze_on_stfDone/1 -> pipeline_delay29/1
  Logical Operator3/1 -> Logical Operator4/3
  Logical Operator/1 -> Logical Operator4/1
